simulink model "simulinkModel"  (R2024b)
settings: Solver=VariableStepAuto  StartTime=0.0  StopTime=10.0  RelTol=1e-3
undefined symbols (not defined in the file): c, d, J
settings Model: Creator=antou  LastModifiedBy=antou

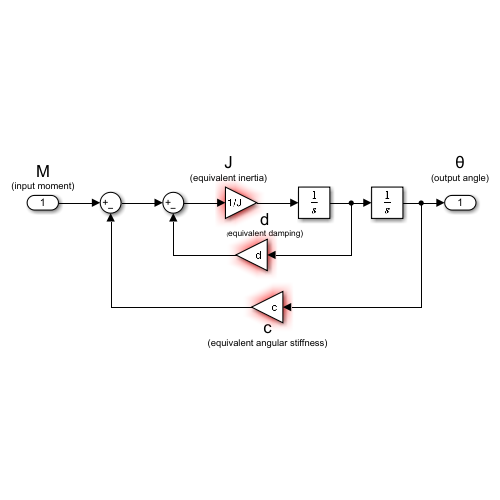
[thumbnail: Simulink's stored preview of the top-level diagram]
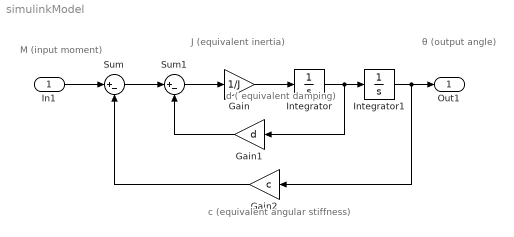
== system simulinkModel ==
  note: M
      | (input moment)
  note: d
      | ( equivalent damping)
  note: c
      | (equivalent angular stiffness)
  note: J
      | (equivalent inertia)
  note: θ
      | (output angle)
  In1 : Inport
  Gain : Gain  Gain=1/J
  Gain1 : Gain  Gain=d
  Gain2 : Gain  Gain=c
  Integrator : Integrator
  Integrator1 : Integrator
  Sum : Sum  Inputs=|+-
  Sum1 : Sum  Inputs=|+-
  Out1 : Outport
  wires:
  In1/1 -> Sum/1
  Gain/1 -> Integrator/1
  Integrator/1 -> Gain1/1, Integrator1/1
  Integrator1/1 -> Gain2/1, Out1/1
  Sum/1 -> Sum1/1
  Sum1/1 -> Gain/1
  Gain1/1 -> Sum1/2
  Gain2/1 -> Sum/2
